simulink library "csu_pwm_pwpf_logic_lib"  (R2015b)
settings: Solver=ode45  StartTime=0.0  StopTime=10.0  RelTol=1e-3
undefined symbols (not defined in the file or in its folder): DiscIntNeverNeededParam
undefined symbols (not defined in the file): ltg_pwpf_accel_err_km, ltg_pwpf_accel_integ_tm, ltg_pwpf_trigger_off_alpha, ltg_pwpf_trigger_on_alpha
libraries: util_info_lib x1
settings Model: Creator=Dan Wibben  LastModifiedBy=jimkaidy
settings DataIOCC: SaveFormat=Array  SignalLoggingSaveFormat=ModelDataLogs
settings OptimizationCC: ExpressionDepthLimit=2147483647
settings DebuggingCC: UnderspecifiedInitializationDetection=Classic  MergeDetectMultiDrivingBlocksExec=none  SolverPrmCheckMsg=warning  FcnCallInpInsideContextMsg=UseLocalSettings  StateNameClashWarn=warning  StrictBusMsg=Warning
settings HardwareCC: ProdBitPerPointer=32  ProdLargestAtomicFloat=None  ProdIntDivRoundTo=Undefined  ProdEndianess=Unspecified  ProdWordSize=32  ProdHWDeviceType=32-bit Generic
settings GRTTargetCC: GeneratePreprocessorConditionals=Disable all  CombineOutputUpdateFcns=off  GRTInterface=on
settings ConfigComp: CovModelRefEnable=Off  CovSFcnEnable=off

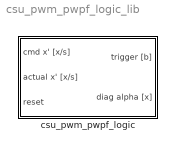
== system csu_pwm_pwpf_logic_lib ==
  csu_pwm_pwpf_logic : Subsystem  mask{Km=ltg_pwpf_accel_err_km, Tm=ltg_pwpf_accel_integ_tm, dt=-1, trigger_on=ltg_pwpf_trigger_on_alpha, trigger_off=ltg_pwpf_trigger_off_alpha}
      mask prompts: trigger_on "Trigger on v"; trigger_off "Trigger off v"

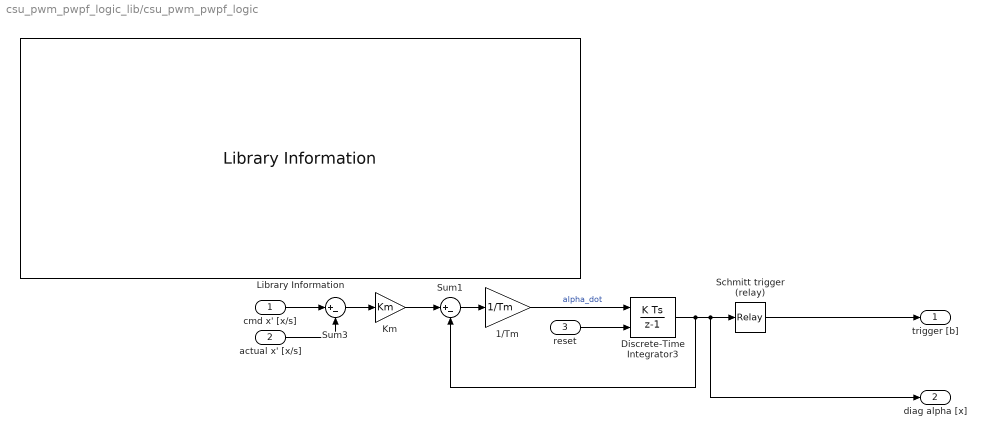
== system csu_pwm_pwpf_logic_lib/csu_pwm_pwpf_logic ==
  cmd x' [x/s] : Inport
  actual x' [x/s] : Inport  Port=2
  reset : Inport  Port=3
  1/Tm : Gain  Gain=1/Tm
  Discrete-Time Integrator3 : DiscreteIntegrator  ExternalReset=rising  SampleTime=dt  ICPrevOutput=DiscIntNeverNeededParam  ICPrevScaledInput=DiscIntNeverNeededParam
  Km : Gain  Gain=Km
  Library Information : util_info_lib/Library Information  owner='NONE'
  Schmitt trigger (relay) : Relay  OnSwitchValue=trigger_on  OffSwitchValue=trigger_off  SampleTime=dt
  Sum1 : Sum  Inputs=|+-
  Sum3 : Sum  Inputs=|+-
  trigger [b] : Outport
  diag alpha [x] : Outport  Port=2
  wires:
  reset/1 -> Discrete-Time Integrator3/2
  Discrete-Time Integrator3/1 -> Sum1/2, Schmitt trigger (relay)/1, diag alpha [x]/1
  actual x' [x/s]/1 -> Sum3/2
  cmd x' [x/s]/1 -> Sum3/1
  Sum3/1 -> Km/1
  Km/1 -> Sum1/1
  Sum1/1 -> 1/Tm/1
  1/Tm/1 -> Discrete-Time Integrator3/1  "alpha_dot"
  Schmitt trigger (relay)/1 -> trigger [b]/1
